simulink model "MSBR_Plant"  (R2021b)
settings: Solver=ode45  StartTime=0.0  StopTime=sim_time  MaxStep=ts_max  RelTol=1e-4
values from neighbouring files (symbols this model uses):
  a_1 = 8.7292e-2/wilson_ratio    (= 0.0087292)    [Whole_Plant_Cool_Pump_Accident_script.m]    (also in Whole_Plant_Fert_Pump_Accident_script.m; Whole_Plant_Fuel_Pump_Accident.m; Whole_Plant_Fuel_Pump_Accident_script.m; Whole_Plant_Reactivity_Accident.m)
  a_2 = 7.3787e-4/wilson_ratio    (= 7.3787e-05)    [Whole_Plant_Cool_Pump_Accident_script.m]    (also in Whole_Plant_Fert_Pump_Accident_script.m; Whole_Plant_Fuel_Pump_Accident.m; Whole_Plant_Fuel_Pump_Accident_script.m; Whole_Plant_Reactivity_Accident.m)
  a_b = 1.656e-5    (= 1.656e-05)    [Whole_Plant_Cool_Pump_Accident_script.m]    (also in Whole_Plant_Fert_Pump_Accident_script.m; Whole_Plant_Fuel_Pump_Accident.m; Whole_Plant_Fuel_Pump_Accident_script.m; Whole_Plant_Reactivity_Accident.m)
  a_f = -8.172e-5    (= -8.172e-05)    [Whole_Plant_Cool_Pump_Accident_script.m]    (also in Whole_Plant_Fert_Pump_Accident_script.m; Whole_Plant_Fuel_Pump_Accident.m; Whole_Plant_Fuel_Pump_Accident_script.m; Whole_Plant_Reactivity_Accident.m)
  a_g = 2.016e-5    (= 2.016e-05)    [Whole_Plant_Cool_Pump_Accident_script.m]    (also in Whole_Plant_Fert_Pump_Accident_script.m; Whole_Plant_Fuel_Pump_Accident.m; Whole_Plant_Fuel_Pump_Accident_script.m; Whole_Plant_Reactivity_Accident.m)
  A_s = pi()*((D_OTSG_i^2)/4) - A_w_OTSG - A_p_OTSG    [Whole_Plant_Cool_Pump_Accident_script.m]    (also in Whole_Plant_Fert_Pump_Accident_script.m; Whole_Plant_Fuel_Pump_Accident.m; Whole_Plant_Fuel_Pump_Accident_script.m; Whole_Plant_Reactivity_Accident.m)
  alpha_co = 316.2    [Whole_Plant_Cool_Pump_Accident_script.m]    (also in Whole_Plant_Fert_Pump_Accident_script.m; Whole_Plant_Fuel_Pump_Accident.m; Whole_Plant_Fuel_Pump_Accident_script.m; Whole_Plant_Reactivity_Accident.m)
  beta = [2.290e-04, 8.320e-04, 7.100e-04, 8.520e-04, 1.710e-04, 1.020e-04]    [Whole_Plant_Cool_Pump_Accident_script.m]    (also in Whole_Plant_Fert_Pump_Accident_script.m; Whole_Plant_Fuel_Pump_Accident.m; Whole_Plant_Fuel_Pump_Accident_script.m; Whole_Plant_Reactivity_Accident.m)
  beta_co = 68.0958    [Whole_Plant_Cool_Pump_Accident_script.m]    (also in Whole_Plant_Fert_Pump_Accident_script.m; Whole_Plant_Fuel_Pump_Accident.m; Whole_Plant_Fuel_Pump_Accident_script.m; Whole_Plant_Reactivity_Accident.m)
  beta_t = sum(beta)    [Whole_Plant_Cool_Pump_Accident_script.m]    (also in Whole_Plant_Fert_Pump_Accident_script.m; Whole_Plant_Fuel_Pump_Accident.m; Whole_Plant_Fuel_Pump_Accident_script.m; Whole_Plant_Reactivity_Accident.m)
  C_nc_X_A_nc = 12.8    [Whole_Plant_Cool_Pump_Accident_script.m]    (also in Whole_Plant_Fert_Pump_Accident_script.m; Whole_Plant_Fuel_Pump_Accident.m; Whole_Plant_Fuel_Pump_Accident_script.m; Whole_Plant_Reactivity_Accident.m)
  C_pcw = 0.0042    [Whole_Plant_Cool_Pump_Accident_script.m]    (also in Whole_Plant_Fert_Pump_Accident_script.m; Whole_Plant_Fuel_Pump_Accident.m; Whole_Plant_Fuel_Pump_Accident_script.m; Whole_Plant_Reactivity_Accident.m)
  C_rh_X_A_rh = 33    [Whole_Plant_Cool_Pump_Accident_script.m]    (also in Whole_Plant_Fert_Pump_Accident_script.m; Whole_Plant_Fuel_Pump_Accident.m; Whole_Plant_Fuel_Pump_Accident_script.m; Whole_Plant_Reactivity_Accident.m)
  C_v = 0.84    [Whole_Plant_Cool_Pump_Accident_script.m]    (also in Whole_Plant_Fert_Pump_Accident_script.m; Whole_Plant_Fuel_Pump_Accident.m; Whole_Plant_Fuel_Pump_Accident_script.m; Whole_Plant_Reactivity_Accident.m)
  ce1 = 1.2471e-07    [Whole_Plant_Cool_Pump_Accident_script.m]    (also in Whole_Plant_Fert_Pump_Accident_script.m; Whole_Plant_Fuel_Pump_Accident.m; Whole_Plant_Fuel_Pump_Accident_script.m; Whole_Plant_Reactivity_Accident.m)
  ce2 = 5.3816e-14    [Whole_Plant_Cool_Pump_Accident_script.m]    (also in Whole_Plant_Fert_Pump_Accident_script.m; Whole_Plant_Fuel_Pump_Accident.m; Whole_Plant_Fuel_Pump_Accident_script.m; Whole_Plant_Reactivity_Accident.m)
  ce3 = 3.3721e-08    [Whole_Plant_Cool_Pump_Accident_script.m]    (also in Whole_Plant_Fert_Pump_Accident_script.m; Whole_Plant_Fuel_Pump_Accident.m; Whole_Plant_Fuel_Pump_Accident_script.m; Whole_Plant_Reactivity_Accident.m)
  Cp_fw = XSteam('Cp_pT',P_set*10,T_fw)/1000    [Whole_Plant_Cool_Pump_Accident_script.m]    (also in Whole_Plant_Fert_Pump_Accident_script.m; Whole_Plant_Fuel_Pump_Accident.m; Whole_Plant_Fuel_Pump_Accident_script.m; Whole_Plant_Reactivity_Accident.m)
  Cp_p = Cp_sec    (= 0.001716588)    [Whole_Plant_Cool_Pump_Accident_script.m]    (also in Whole_Plant_Fert_Pump_Accident_script.m; Whole_Plant_Fuel_Pump_Accident.m; Whole_Plant_Fuel_Pump_Accident_script.m; Whole_Plant_Reactivity_Accident.m)
  Cp_rh = 0.0021520    (= 0.002152)    [Whole_Plant_Cool_Pump_Accident_script.m]    (also in Whole_Plant_Fert_Pump_Accident_script.m; Whole_Plant_Fuel_Pump_Accident.m; Whole_Plant_Fuel_Pump_Accident_script.m; Whole_Plant_Reactivity_Accident.m)
  Cp_s = XSteam('Cp_pT',P_s*10,T_s)/1000    [Whole_Plant_Cool_Pump_Accident_script.m]    (also in Whole_Plant_Fert_Pump_Accident_script.m; Whole_Plant_Fuel_Pump_Accident.m; Whole_Plant_Fuel_Pump_Accident_script.m; Whole_Plant_Reactivity_Accident.m)
  Cp_sc = XSteam('Cp_pT',P_set*10,T_sc2)/1000    [Whole_Plant_Cool_Pump_Accident_script.m]    (also in Whole_Plant_Fert_Pump_Accident_script.m; Whole_Plant_Fuel_Pump_Accident.m; Whole_Plant_Fuel_Pump_Accident_script.m; Whole_Plant_Reactivity_Accident.m)
  Cp_w = 468.992e-6    (= 0.000468992)    [Whole_Plant_Cool_Pump_Accident_script.m]    (also in Whole_Plant_Fert_Pump_Accident_script.m; Whole_Plant_Fuel_Pump_Accident.m; Whole_Plant_Fuel_Pump_Accident_script.m; Whole_Plant_Reactivity_Accident.m)
  D_it = D_ot-2*T_th    (= 0.014147)    [Whole_Plant_Cool_Pump_Accident_script.m]    (also in Whole_Plant_Fert_Pump_Accident_script.m; Whole_Plant_Fuel_Pump_Accident.m; Whole_Plant_Fuel_Pump_Accident_script.m; Whole_Plant_Reactivity_Accident.m)
  D_ot = 0.015875    [Whole_Plant_Cool_Pump_Accident_script.m]    (also in Whole_Plant_Fert_Pump_Accident_script.m; Whole_Plant_Fuel_Pump_Accident.m; Whole_Plant_Fuel_Pump_Accident_script.m; Whole_Plant_Reactivity_Accident.m)
  dHs_dPs = c(1)    [Whole_Plant_Cool_Pump_Accident_script.m]    (also in Whole_Plant_Fert_Pump_Accident_script.m; Whole_Plant_Fuel_Pump_Accident.m; Whole_Plant_Fuel_Pump_Accident_script.m; Whole_Plant_Reactivity_Accident.m)
  eta_hp_isen = 0.861    [Whole_Plant_Cool_Pump_Accident_script.m]    (also in Whole_Plant_Fert_Pump_Accident_script.m; Whole_Plant_Fuel_Pump_Accident.m; Whole_Plant_Fuel_Pump_Accident_script.m; Whole_Plant_Reactivity_Accident.m)
  eta_lp_isen = 0.861    [Whole_Plant_Cool_Pump_Accident_script.m]    (also in Whole_Plant_Fert_Pump_Accident_script.m; Whole_Plant_Fuel_Pump_Accident.m; Whole_Plant_Fuel_Pump_Accident_script.m; Whole_Plant_Reactivity_Accident.m)
  gamma_I = 5.1135e-2    (= 0.051135)    [Whole_Plant_Cool_Pump_Accident_script.m]    (also in Whole_Plant_Fert_Pump_Accident_script.m; Whole_Plant_Fuel_Pump_Accident.m; Whole_Plant_Fuel_Pump_Accident_script.m; Whole_Plant_Reactivity_Accident.m)
  gamma_Xe = 1.1628e-2    (= 0.011628)    [Whole_Plant_Cool_Pump_Accident_script.m]    (also in Whole_Plant_Fert_Pump_Accident_script.m; Whole_Plant_Fuel_Pump_Accident.m; Whole_Plant_Fuel_Pump_Accident_script.m; Whole_Plant_Reactivity_Accident.m)
  H_co0 = 0.149    [Whole_Plant_Cool_Pump_Accident_script.m]    (also in Whole_Plant_Fert_Pump_Accident_script.m; Whole_Plant_Fuel_Pump_Accident.m; Whole_Plant_Fuel_Pump_Accident_script.m; Whole_Plant_Reactivity_Accident.m)
  H_f_co0 = 0.149    [Whole_Plant_Cool_Pump_Accident_script.m]    (also in Whole_Plant_Fert_Pump_Accident_script.m; Whole_Plant_Fuel_Pump_Accident.m; Whole_Plant_Fuel_Pump_Accident_script.m; Whole_Plant_Reactivity_Accident.m)
  H_fg_co0 = 2.35    [Whole_Plant_Cool_Pump_Accident_script.m]    (also in Whole_Plant_Fert_Pump_Accident_script.m; Whole_Plant_Fuel_Pump_Accident.m; Whole_Plant_Fuel_Pump_Accident_script.m; Whole_Plant_Reactivity_Accident.m)
  H_fgrh0 = (XSteam('hV_p', P_s*1e1) - XSteam('hL_p', P_s*1e1))/1e3    [Whole_Plant_Cool_Pump_Accident_script.m]    (also in Whole_Plant_Fert_Pump_Accident_script.m; Whole_Plant_Fuel_Pump_Accident.m; Whole_Plant_Fuel_Pump_Accident_script.m; Whole_Plant_Reactivity_Accident.m)
  H_frh0 = XSteam('hL_p', P_s*1e1)/1e3    [Whole_Plant_Cool_Pump_Accident_script.m]    (also in Whole_Plant_Fert_Pump_Accident_script.m; Whole_Plant_Fuel_Pump_Accident.m; Whole_Plant_Fuel_Pump_Accident_script.m; Whole_Plant_Reactivity_Accident.m)
  h_fwh1 = 0.5927    [Whole_Plant_Cool_Pump_Accident_script.m]    (also in Whole_Plant_Fert_Pump_Accident_script.m; Whole_Plant_Fuel_Pump_Accident.m; Whole_Plant_Fuel_Pump_Accident_script.m; Whole_Plant_Reactivity_Accident.m)
  H_fwh10 = 0.46009    [Whole_Plant_Cool_Pump_Accident_script.m]    (also in Whole_Plant_Fert_Pump_Accident_script.m; Whole_Plant_Fuel_Pump_Accident.m; Whole_Plant_Fuel_Pump_Accident_script.m; Whole_Plant_Reactivity_Accident.m)
  h_fwh2 = 1.230803    [Whole_Plant_Cool_Pump_Accident_script.m]    (also in Whole_Plant_Fert_Pump_Accident_script.m; Whole_Plant_Fuel_Pump_Accident.m; Whole_Plant_Fuel_Pump_Accident_script.m; Whole_Plant_Reactivity_Accident.m)
  H_fwh20 = 0.6784    [Whole_Plant_Cool_Pump_Accident_script.m]    (also in Whole_Plant_Fert_Pump_Accident_script.m; Whole_Plant_Fuel_Pump_Accident.m; Whole_Plant_Fuel_Pump_Accident_script.m; Whole_Plant_Reactivity_Accident.m)
  H_grh0 = 2.8029    [Whole_Plant_Cool_Pump_Accident_script.m]    (also in Whole_Plant_Fert_Pump_Accident_script.m; Whole_Plant_Fuel_Pump_Accident.m; Whole_Plant_Fuel_Pump_Accident_script.m; Whole_Plant_Reactivity_Accident.m)
  H_hp_isen0 = 2.5111    [Whole_Plant_Cool_Pump_Accident_script.m]    (also in Whole_Plant_Fert_Pump_Accident_script.m; Whole_Plant_Fuel_Pump_Accident.m; Whole_Plant_Fuel_Pump_Accident_script.m; Whole_Plant_Reactivity_Accident.m)
  H_hpt_out = 2.6201    [Whole_Plant_Cool_Pump_Accident_script.m]    (also in Whole_Plant_Fert_Pump_Accident_script.m; Whole_Plant_Fuel_Pump_Accident.m; Whole_Plant_Fuel_Pump_Accident_script.m; Whole_Plant_Reactivity_Accident.m)
  H_lp_isen = 958.4*1054.35e-6/0.45359237    (= 2.22774699671)    [Whole_Plant_Cool_Pump_Accident_script.m]    (also in Whole_Plant_Fert_Pump_Accident_script.m; Whole_Plant_Fuel_Pump_Accident.m; Whole_Plant_Fuel_Pump_Accident_script.m; Whole_Plant_Reactivity_Accident.m)
  H_lpt_out = 2.3089    [Whole_Plant_Cool_Pump_Accident_script.m]    (also in Whole_Plant_Fert_Pump_Accident_script.m; Whole_Plant_Fuel_Pump_Accident.m; Whole_Plant_Fuel_Pump_Accident_script.m; Whole_Plant_Reactivity_Accident.m)
  H_nc = XSteam('h_pT', P_s*10, T_s)/1000    [Whole_Plant_Cool_Pump_Accident_script.m]    (also in Whole_Plant_Fert_Pump_Accident_script.m; Whole_Plant_Fuel_Pump_Accident.m; Whole_Plant_Fuel_Pump_Accident_script.m; Whole_Plant_Reactivity_Accident.m)
  h_pw = h_s    (= 0.02555)    [Whole_Plant_Cool_Pump_Accident_script.m]    (also in Whole_Plant_Fert_Pump_Accident_script.m; Whole_Plant_Fuel_Pump_Accident.m; Whole_Plant_Fuel_Pump_Accident_script.m; Whole_Plant_Reactivity_Accident.m)
  H_rh = 2.8115    [Whole_Plant_Cool_Pump_Accident_script.m]    (also in Whole_Plant_Fert_Pump_Accident_script.m; Whole_Plant_Fuel_Pump_Accident.m; Whole_Plant_Fuel_Pump_Accident_script.m; Whole_Plant_Reactivity_Accident.m)
  h_wb = 13349.334646671E-6    (= 0.0133493346467)    [Whole_Plant_Cool_Pump_Accident_script.m]    (also in Whole_Plant_Fert_Pump_Accident_script.m; Whole_Plant_Fuel_Pump_Accident.m; Whole_Plant_Fuel_Pump_Accident_script.m; Whole_Plant_Reactivity_Accident.m)
  h_ws = 5732.378387768E-6    (= 0.00573237838777)    [Whole_Plant_Cool_Pump_Accident_script.m]    (also in Whole_Plant_Fert_Pump_Accident_script.m; Whole_Plant_Fuel_Pump_Accident.m; Whole_Plant_Fuel_Pump_Accident_script.m; Whole_Plant_Reactivity_Accident.m)
  h_wsc = 8385.005556375E-6    (= 0.00838500555638)    [Whole_Plant_Cool_Pump_Accident_script.m]    (also in Whole_Plant_Fert_Pump_Accident_script.m; Whole_Plant_Fuel_Pump_Accident.m; Whole_Plant_Fuel_Pump_Accident_script.m; Whole_Plant_Reactivity_Accident.m)
  hA_bg = A_fert*h_bg    (= 2.76411813627)    [Whole_Plant_Cool_Pump_Accident_script.m]    (also in Whole_Plant_Fert_Pump_Accident_script.m; Whole_Plant_Fuel_Pump_Accident.m; Whole_Plant_Fuel_Pump_Accident_script.m; Whole_Plant_Reactivity_Accident.m)
  hA_co0 = 140    [Whole_Plant_Cool_Pump_Accident_script.m]    (also in Whole_Plant_Fert_Pump_Accident_script.m; Whole_Plant_Fuel_Pump_Accident.m; Whole_Plant_Fuel_Pump_Accident_script.m; Whole_Plant_Reactivity_Accident.m)
  hA_fg_dn = h_fg*A_fuel_down    [Whole_Plant_Cool_Pump_Accident_script.m]    (also in Whole_Plant_Fert_Pump_Accident_script.m; Whole_Plant_Fuel_Pump_Accident.m; Whole_Plant_Fuel_Pump_Accident_script.m; Whole_Plant_Reactivity_Accident.m)
  hA_fg_up = h_fg*A_fuel_up    [Whole_Plant_Cool_Pump_Accident_script.m]    (also in Whole_Plant_Fert_Pump_Accident_script.m; Whole_Plant_Fuel_Pump_Accident.m; Whole_Plant_Fuel_Pump_Accident_script.m; Whole_Plant_Reactivity_Accident.m)
  hA_p_bhx1 = [h_pb*A_pbhx/2,h_pb*A_pbhx/2]    [Whole_Plant_Cool_Pump_Accident_script.m]    (also in Whole_Plant_Fert_Pump_Accident_script.m; Whole_Plant_Fuel_Pump_Accident.m; Whole_Plant_Fuel_Pump_Accident_script.m; Whole_Plant_Reactivity_Accident.m)
  hA_p_bhx2 = hA_p_bhx1    [Whole_Plant_Cool_Pump_Accident_script.m]    (also in Whole_Plant_Fert_Pump_Accident_script.m; Whole_Plant_Fuel_Pump_Accident.m; Whole_Plant_Fuel_Pump_Accident_script.m; Whole_Plant_Reactivity_Accident.m)
  hA_p_bhx3 = hA_p_bhx1    [Whole_Plant_Cool_Pump_Accident_script.m]    (also in Whole_Plant_Fert_Pump_Accident_script.m; Whole_Plant_Fuel_Pump_Accident.m; Whole_Plant_Fuel_Pump_Accident_script.m; Whole_Plant_Reactivity_Accident.m)
  hA_p_bhx4 = hA_p_bhx1    [Whole_Plant_Cool_Pump_Accident_script.m]    (also in Whole_Plant_Fert_Pump_Accident_script.m; Whole_Plant_Fuel_Pump_Accident.m; Whole_Plant_Fuel_Pump_Accident_script.m; Whole_Plant_Reactivity_Accident.m)
  hA_p_fhx1 = [h_p*A_pfhx_dn/2,h_p*A_pfhx_dn/2,h_p*A_pfhx_up/2,h_p*A_pfhx_up/2]    [Whole_Plant_Cool_Pump_Accident_script.m]    (also in Whole_Plant_Fert_Pump_Accident_script.m; Whole_Plant_Fuel_Pump_Accident.m; Whole_Plant_Fuel_Pump_Accident_script.m; Whole_Plant_Reactivity_Accident.m)
  hA_p_fhx2 = hA_p_fhx1    [Whole_Plant_Cool_Pump_Accident_script.m]    (also in Whole_Plant_Fert_Pump_Accident_script.m; Whole_Plant_Fuel_Pump_Accident.m; Whole_Plant_Fuel_Pump_Accident_script.m; Whole_Plant_Reactivity_Accident.m)
  hA_p_fhx3 = hA_p_fhx1    [Whole_Plant_Cool_Pump_Accident_script.m]    (also in Whole_Plant_Fert_Pump_Accident_script.m; Whole_Plant_Fuel_Pump_Accident.m; Whole_Plant_Fuel_Pump_Accident_script.m; Whole_Plant_Reactivity_Accident.m)
  hA_p_fhx4 = hA_p_fhx1    [Whole_Plant_Cool_Pump_Accident_script.m]    (also in Whole_Plant_Fert_Pump_Accident_script.m; Whole_Plant_Fuel_Pump_Accident.m; Whole_Plant_Fuel_Pump_Accident_script.m; Whole_Plant_Reactivity_Accident.m)
  hA_s_bhx1 = [h_sb*A_sbhx/2,h_sb*A_sbhx/2]    [Whole_Plant_Cool_Pump_Accident_script.m]    (also in Whole_Plant_Fert_Pump_Accident_script.m; Whole_Plant_Fuel_Pump_Accident.m; Whole_Plant_Fuel_Pump_Accident_script.m; Whole_Plant_Reactivity_Accident.m)
  hA_s_bhx2 = hA_s_bhx1    [Whole_Plant_Cool_Pump_Accident_script.m]    (also in Whole_Plant_Fert_Pump_Accident_script.m; Whole_Plant_Fuel_Pump_Accident.m; Whole_Plant_Fuel_Pump_Accident_script.m; Whole_Plant_Reactivity_Accident.m)
  hA_s_bhx3 = hA_s_bhx1    [Whole_Plant_Cool_Pump_Accident_script.m]    (also in Whole_Plant_Fert_Pump_Accident_script.m; Whole_Plant_Fuel_Pump_Accident.m; Whole_Plant_Fuel_Pump_Accident_script.m; Whole_Plant_Reactivity_Accident.m)
  hA_s_bhx4 = hA_s_bhx1    [Whole_Plant_Cool_Pump_Accident_script.m]    (also in Whole_Plant_Fert_Pump_Accident_script.m; Whole_Plant_Fuel_Pump_Accident.m; Whole_Plant_Fuel_Pump_Accident_script.m; Whole_Plant_Reactivity_Accident.m)
  hA_s_fhx1 = [h_s*A_sfhx_up/2,h_s*A_sfhx_up/2,h_s*A_sfhx_dn/2,h_s*A_sfhx_dn/2]    [Whole_Plant_Cool_Pump_Accident_script.m]    (also in Whole_Plant_Fert_Pump_Accident_script.m; Whole_Plant_Fuel_Pump_Accident.m; Whole_Plant_Fuel_Pump_Accident_script.m; Whole_Plant_Reactivity_Accident.m)
  hA_s_fhx2 = hA_s_fhx1    [Whole_Plant_Cool_Pump_Accident_script.m]    (also in Whole_Plant_Fert_Pump_Accident_script.m; Whole_Plant_Fuel_Pump_Accident.m; Whole_Plant_Fuel_Pump_Accident_script.m; Whole_Plant_Reactivity_Accident.m)
  hA_s_fhx3 = hA_s_fhx1    [Whole_Plant_Cool_Pump_Accident_script.m]    (also in Whole_Plant_Fert_Pump_Accident_script.m; Whole_Plant_Fuel_Pump_Accident.m; Whole_Plant_Fuel_Pump_Accident_script.m; Whole_Plant_Reactivity_Accident.m)
  hA_s_fhx4 = hA_s_fhx1    [Whole_Plant_Cool_Pump_Accident_script.m]    (also in Whole_Plant_Fert_Pump_Accident_script.m; Whole_Plant_Fuel_Pump_Accident.m; Whole_Plant_Fuel_Pump_Accident_script.m; Whole_Plant_Reactivity_Accident.m)
  I_0 = gamma_I*Sigma_f_msbr*phi_0/lam_I    (= 1.30000734126e+17)    [Whole_Plant_Cool_Pump_Accident_script.m]    (also in Whole_Plant_Fert_Pump_Accident_script.m; Whole_Plant_Fuel_Pump_Accident.m; Whole_Plant_Fuel_Pump_Accident_script.m; Whole_Plant_Reactivity_Accident.m)
  k_1 = 0.5    [Whole_Plant_Cool_Pump_Accident_script.m]    (also in Whole_Plant_Fert_Pump_Accident_script.m; Whole_Plant_Fuel_Pump_Accident.m; Whole_Plant_Fuel_Pump_Accident_script.m; Whole_Plant_Reactivity_Accident.m)
  K_1 = e(1)    [Whole_Plant_Cool_Pump_Accident_script.m]    (also in Whole_Plant_Fert_Pump_Accident_script.m; Whole_Plant_Fuel_Pump_Accident.m; Whole_Plant_Fuel_Pump_Accident_script.m; Whole_Plant_Reactivity_Accident.m)
  k_1b = 0.5    [Whole_Plant_Cool_Pump_Accident_script.m]    (also in Whole_Plant_Fert_Pump_Accident_script.m; Whole_Plant_Fuel_Pump_Accident.m; Whole_Plant_Fuel_Pump_Accident_script.m; Whole_Plant_Reactivity_Accident.m)
  k_2 = 0.5    [Whole_Plant_Cool_Pump_Accident_script.m]    (also in Whole_Plant_Fert_Pump_Accident_script.m; Whole_Plant_Fuel_Pump_Accident.m; Whole_Plant_Fuel_Pump_Accident_script.m; Whole_Plant_Reactivity_Accident.m)
  k_2b = 0.5    [Whole_Plant_Cool_Pump_Accident_script.m]    (also in Whole_Plant_Fert_Pump_Accident_script.m; Whole_Plant_Fuel_Pump_Accident.m; Whole_Plant_Fuel_Pump_Accident_script.m; Whole_Plant_Reactivity_Accident.m)
  k_3 = 0.5    [Whole_Plant_Cool_Pump_Accident_script.m]    (also in Whole_Plant_Fert_Pump_Accident_script.m; Whole_Plant_Fuel_Pump_Accident.m; Whole_Plant_Fuel_Pump_Accident_script.m; Whole_Plant_Reactivity_Accident.m)
  k_4 = 0.5    [Whole_Plant_Cool_Pump_Accident_script.m]    (also in Whole_Plant_Fert_Pump_Accident_script.m; Whole_Plant_Fuel_Pump_Accident.m; Whole_Plant_Fuel_Pump_Accident_script.m; Whole_Plant_Reactivity_Accident.m)
  K_4 = b(1)    [Whole_Plant_Cool_Pump_Accident_script.m]    (also in Whole_Plant_Fert_Pump_Accident_script.m; Whole_Plant_Fuel_Pump_Accident.m; Whole_Plant_Fuel_Pump_Accident_script.m; Whole_Plant_Reactivity_Accident.m)
  K_5 = a(1)    [Whole_Plant_Cool_Pump_Accident_script.m]    (also in Whole_Plant_Fert_Pump_Accident_script.m; Whole_Plant_Fuel_Pump_Accident.m; Whole_Plant_Fuel_Pump_Accident_script.m; Whole_Plant_Reactivity_Accident.m)
  K_b = d(1)    [Whole_Plant_Cool_Pump_Accident_script.m]    (also in Whole_Plant_Fert_Pump_Accident_script.m; Whole_Plant_Fuel_Pump_Accident.m; Whole_Plant_Fuel_Pump_Accident_script.m; Whole_Plant_Reactivity_Accident.m)
  k_b1 = (K_B/2)/K    (= 0.0089463103122)    [Whole_Plant_Cool_Pump_Accident_script.m]    (also in Whole_Plant_Fert_Pump_Accident_script.m; Whole_Plant_Fuel_Pump_Accident.m; Whole_Plant_Fuel_Pump_Accident_script.m; Whole_Plant_Reactivity_Accident.m)
  k_b2 = k_b1    (= 0.0089463103122)    [Whole_Plant_Cool_Pump_Accident_script.m]    (also in Whole_Plant_Fert_Pump_Accident_script.m; Whole_Plant_Fuel_Pump_Accident.m; Whole_Plant_Fuel_Pump_Accident_script.m; Whole_Plant_Reactivity_Accident.m)
  K_bhp = 0.1634    [Whole_Plant_Cool_Pump_Accident_script.m]    (also in Whole_Plant_Fert_Pump_Accident_script.m; Whole_Plant_Fuel_Pump_Accident.m; Whole_Plant_Fuel_Pump_Accident_script.m; Whole_Plant_Reactivity_Accident.m)
  K_blp = 0.2174    [Whole_Plant_Cool_Pump_Accident_script.m]    (also in Whole_Plant_Fert_Pump_Accident_script.m; Whole_Plant_Fuel_Pump_Accident.m; Whole_Plant_Fuel_Pump_Accident_script.m; Whole_Plant_Reactivity_Accident.m)
  k_f1 = ((1 - K_G - K_B - K_Ba)/4)/K    (= 0.226055463576)    [Whole_Plant_Cool_Pump_Accident_script.m]    (also in Whole_Plant_Fert_Pump_Accident_script.m; Whole_Plant_Fuel_Pump_Accident.m; Whole_Plant_Fuel_Pump_Accident_script.m; Whole_Plant_Reactivity_Accident.m)
  k_f2 = k_f1    (= 0.226055463576)    [Whole_Plant_Cool_Pump_Accident_script.m]    (also in Whole_Plant_Fert_Pump_Accident_script.m; Whole_Plant_Fuel_Pump_Accident.m; Whole_Plant_Fuel_Pump_Accident_script.m; Whole_Plant_Reactivity_Accident.m)
  k_f3 = k_f1    (= 0.226055463576)    [Whole_Plant_Cool_Pump_Accident_script.m]    (also in Whole_Plant_Fert_Pump_Accident_script.m; Whole_Plant_Fuel_Pump_Accident.m; Whole_Plant_Fuel_Pump_Accident_script.m; Whole_Plant_Reactivity_Accident.m)
  k_f4 = k_f1    (= 0.226055463576)    [Whole_Plant_Cool_Pump_Accident_script.m]    (also in Whole_Plant_Fert_Pump_Accident_script.m; Whole_Plant_Fuel_Pump_Accident.m; Whole_Plant_Fuel_Pump_Accident_script.m; Whole_Plant_Reactivity_Accident.m)
  k_g1 = ((K_G*K_fuel)/2)/K    (= 0.0346590586566)    [Whole_Plant_Cool_Pump_Accident_script.m]    (also in Whole_Plant_Fert_Pump_Accident_script.m; Whole_Plant_Fuel_Pump_Accident.m; Whole_Plant_Fuel_Pump_Accident_script.m; Whole_Plant_Reactivity_Accident.m)
  k_g2 = k_g1    (= 0.0346590586566)    [Whole_Plant_Cool_Pump_Accident_script.m]    (also in Whole_Plant_Fert_Pump_Accident_script.m; Whole_Plant_Fuel_Pump_Accident.m; Whole_Plant_Fuel_Pump_Accident_script.m; Whole_Plant_Reactivity_Accident.m)
  k_g3 = (K_G*(1-K_fuel))/K    (= 0.00856740775781)    [Whole_Plant_Cool_Pump_Accident_script.m]    (also in Whole_Plant_Fert_Pump_Accident_script.m; Whole_Plant_Fuel_Pump_Accident.m; Whole_Plant_Fuel_Pump_Accident_script.m; Whole_Plant_Reactivity_Accident.m)
  K_sc = f(1)    [Whole_Plant_Cool_Pump_Accident_script.m]    (also in Whole_Plant_Fert_Pump_Accident_script.m; Whole_Plant_Fuel_Pump_Accident.m; Whole_Plant_Fuel_Pump_Accident_script.m; Whole_Plant_Reactivity_Accident.m)
  L = 22.0    (= 22)    [Whole_Plant_Cool_Pump_Accident_script.m]    (also in Whole_Plant_Fert_Pump_Accident_script.m; Whole_Plant_Fuel_Pump_Accident.m; Whole_Plant_Fuel_Pump_Accident_script.m; Whole_Plant_Reactivity_Accident.m)
  L_b = 1.9    [Whole_Plant_Cool_Pump_Accident_script.m]    (also in Whole_Plant_Fert_Pump_Accident_script.m; Whole_Plant_Fuel_Pump_Accident.m; Whole_Plant_Fuel_Pump_Accident_script.m; Whole_Plant_Reactivity_Accident.m)
  L_s = 16.53    [Whole_Plant_Cool_Pump_Accident_script.m]    (also in Whole_Plant_Fert_Pump_Accident_script.m; Whole_Plant_Fuel_Pump_Accident.m; Whole_Plant_Fuel_Pump_Accident_script.m; Whole_Plant_Reactivity_Accident.m)
  L_sc = L-L_b-L_s    (= 3.57)    [Whole_Plant_Cool_Pump_Accident_script.m]    (also in Whole_Plant_Fert_Pump_Accident_script.m; Whole_Plant_Fuel_Pump_Accident.m; Whole_Plant_Fuel_Pump_Accident_script.m; Whole_Plant_Reactivity_Accident.m)
  Lam = 3.3e-4    (= 0.00033)    [Whole_Plant_Cool_Pump_Accident_script.m]    (also in Whole_Plant_Fert_Pump_Accident_script.m; Whole_Plant_Fuel_Pump_Accident.m; Whole_Plant_Fuel_Pump_Accident_script.m; Whole_Plant_Reactivity_Accident.m)
  lam = [1.260e-02, 3.370e-02, 1.390e-01, 3.250e-01, 1.130e+00, 2.500e+00]    [Whole_Plant_Cool_Pump_Accident_script.m]    (also in Whole_Plant_Fert_Pump_Accident_script.m; Whole_Plant_Fuel_Pump_Accident.m; Whole_Plant_Fuel_Pump_Accident_script.m; Whole_Plant_Reactivity_Accident.m)
  lam_bubl = 2.0e-2    (= 0.02)    [Whole_Plant_Cool_Pump_Accident_script.m]    (also in Whole_Plant_Fert_Pump_Accident_script.m; Whole_Plant_Fuel_Pump_Accident.m; Whole_Plant_Fuel_Pump_Accident_script.m; Whole_Plant_Reactivity_Accident.m)
  lam_I = 2.875e-5    (= 2.875e-05)    [Whole_Plant_Cool_Pump_Accident_script.m]    (also in Whole_Plant_Fert_Pump_Accident_script.m; Whole_Plant_Fuel_Pump_Accident.m; Whole_Plant_Fuel_Pump_Accident_script.m; Whole_Plant_Reactivity_Accident.m)
  lam_Xe = 2.0916e-5    (= 2.0916e-05)    [Whole_Plant_Cool_Pump_Accident_script.m]    (also in Whole_Plant_Fert_Pump_Accident_script.m; Whole_Plant_Fuel_Pump_Accident.m; Whole_Plant_Fuel_Pump_Accident_script.m; Whole_Plant_Reactivity_Accident.m)
  m_bm = (W_b1+W_b2+W_b3+W_b4)*time_mixb    (= 2167.1636)    [Whole_Plant_Cool_Pump_Accident_script.m]    (also in Whole_Plant_Fert_Pump_Accident_script.m; Whole_Plant_Fuel_Pump_Accident.m; Whole_Plant_Fuel_Pump_Accident_script.m; Whole_Plant_Reactivity_Accident.m)
  M_cw = 65000    [Whole_Plant_Cool_Pump_Accident_script.m]    (also in Whole_Plant_Fert_Pump_Accident_script.m; Whole_Plant_Fuel_Pump_Accident.m; Whole_Plant_Fuel_Pump_Accident_script.m; Whole_Plant_Reactivity_Accident.m)
  m_fm = (W_f1+W_f2+W_f3+W_f4)*time_mixf    (= 5443.108)    [Whole_Plant_Cool_Pump_Accident_script.m]    (also in Whole_Plant_Fert_Pump_Accident_script.m; Whole_Plant_Fuel_Pump_Accident.m; Whole_Plant_Fuel_Pump_Accident_script.m; Whole_Plant_Reactivity_Accident.m)
  M_hw0 = 10000    [Whole_Plant_Cool_Pump_Accident_script.m]    (also in Whole_Plant_Fert_Pump_Accident_script.m; Whole_Plant_Fuel_Pump_Accident.m; Whole_Plant_Fuel_Pump_Accident_script.m; Whole_Plant_Reactivity_Accident.m)
  m_sm = (W_s1+W_s2+W_s3+W_s4)*time_mixs    (= 8467.056)    [Whole_Plant_Cool_Pump_Accident_script.m]    (also in Whole_Plant_Fert_Pump_Accident_script.m; Whole_Plant_Fuel_Pump_Accident.m; Whole_Plant_Fuel_Pump_Accident_script.m; Whole_Plant_Reactivity_Accident.m)
  M_stm = 0.018    [Whole_Plant_Cool_Pump_Accident_script.m]    (also in Whole_Plant_Fert_Pump_Accident_script.m; Whole_Plant_Fuel_Pump_Accident.m; Whole_Plant_Fuel_Pump_Accident_script.m; Whole_Plant_Reactivity_Accident.m)
  mcp_b1 = mass_bn*Cp_b    (= 4.17494922705)    [Whole_Plant_Cool_Pump_Accident_script.m]    (also in Whole_Plant_Fert_Pump_Accident_script.m; Whole_Plant_Fuel_Pump_Accident.m; Whole_Plant_Fuel_Pump_Accident_script.m; Whole_Plant_Reactivity_Accident.m)
  mcp_b2 = mcp_b1    (= 4.17494922705)    [Whole_Plant_Cool_Pump_Accident_script.m]    (also in Whole_Plant_Fert_Pump_Accident_script.m; Whole_Plant_Fuel_Pump_Accident.m; Whole_Plant_Fuel_Pump_Accident_script.m; Whole_Plant_Reactivity_Accident.m)
  mcp_f1 = mass_fn*Cp_f    (= 5.5019469141)    [Whole_Plant_Cool_Pump_Accident_script.m]    (also in Whole_Plant_Fert_Pump_Accident_script.m; Whole_Plant_Fuel_Pump_Accident.m; Whole_Plant_Fuel_Pump_Accident_script.m; Whole_Plant_Reactivity_Accident.m)
  mcp_f2 = mass_fn*Cp_f    (= 5.5019469141)    [Whole_Plant_Cool_Pump_Accident_script.m]    (also in Whole_Plant_Fert_Pump_Accident_script.m; Whole_Plant_Fuel_Pump_Accident.m; Whole_Plant_Fuel_Pump_Accident_script.m; Whole_Plant_Reactivity_Accident.m)
  mcp_f3 = mass_fn*Cp_f    (= 5.5019469141)    [Whole_Plant_Cool_Pump_Accident_script.m]    (also in Whole_Plant_Fert_Pump_Accident_script.m; Whole_Plant_Fuel_Pump_Accident.m; Whole_Plant_Fuel_Pump_Accident_script.m; Whole_Plant_Reactivity_Accident.m)
  mcp_f4 = mass_fn*Cp_f    (= 5.5019469141)    [Whole_Plant_Cool_Pump_Accident_script.m]    (also in Whole_Plant_Fert_Pump_Accident_script.m; Whole_Plant_Fuel_Pump_Accident.m; Whole_Plant_Fuel_Pump_Accident_script.m; Whole_Plant_Reactivity_Accident.m)
  mcp_g1 = (mass_grap*Cp_g)*K_fuel/2    (= 32.9814988203)    [Whole_Plant_Cool_Pump_Accident_script.m]    (also in Whole_Plant_Fert_Pump_Accident_script.m; Whole_Plant_Fuel_Pump_Accident.m; Whole_Plant_Fuel_Pump_Accident_script.m; Whole_Plant_Reactivity_Accident.m)
  mcp_g2 = mcp_g1    (= 32.9814988203)    [Whole_Plant_Cool_Pump_Accident_script.m]    (also in Whole_Plant_Fert_Pump_Accident_script.m; Whole_Plant_Fuel_Pump_Accident.m; Whole_Plant_Fuel_Pump_Accident_script.m; Whole_Plant_Reactivity_Accident.m)
  mcp_g3 = (mass_grap*Cp_g)*(1-K_fuel)    (= 8.15273004546)    [Whole_Plant_Cool_Pump_Accident_script.m]    (also in Whole_Plant_Fert_Pump_Accident_script.m; Whole_Plant_Fuel_Pump_Accident.m; Whole_Plant_Fuel_Pump_Accident_script.m; Whole_Plant_Reactivity_Accident.m)
  mcp_p_bhx1 = mp_bhx1*Cp_b    [Whole_Plant_Cool_Pump_Accident_script.m]    (also in Whole_Plant_Fert_Pump_Accident_script.m; Whole_Plant_Fuel_Pump_Accident.m; Whole_Plant_Fuel_Pump_Accident_script.m; Whole_Plant_Reactivity_Accident.m)
  mcp_p_bhx2 = mp_bhx2*Cp_b    [Whole_Plant_Cool_Pump_Accident_script.m]    (also in Whole_Plant_Fert_Pump_Accident_script.m; Whole_Plant_Fuel_Pump_Accident.m; Whole_Plant_Fuel_Pump_Accident_script.m; Whole_Plant_Reactivity_Accident.m)
  mcp_p_bhx3 = mp_bhx3*Cp_b    [Whole_Plant_Cool_Pump_Accident_script.m]    (also in Whole_Plant_Fert_Pump_Accident_script.m; Whole_Plant_Fuel_Pump_Accident.m; Whole_Plant_Fuel_Pump_Accident_script.m; Whole_Plant_Reactivity_Accident.m)
  ... (+213 more)
undefined symbols (not defined in the file or in its folder): C0, H_con_table, H_convap_table, H_rh_table, H_rh_table1, H_rh_table2, H_rhvap_table, H_s_table, H_table, P_con_table, P_nc_table, P_rh_table, P_rh_table1, pres_table, rho_rh_table, rho_table, SV_nc_table, SVf_nc_table, temp_table
(part 3 of 13)

== system MSBR_Plant/Nuclear Steam Supply System (NSSS)/MSBR ==
  In Bus Element2 : Inport  PortName=Core Inlet  Element=Fuel Heat Transfer Fraction
  In Bus Element : Inport  PortName=Core Inlet  Element=Hx Fuel Outlet Temp
  In Bus Element1 : Inport  PortName=Core Inlet  Element=Fuel Flow Fraction
  In Bus Element4 : Inport  PortName=Core Inlet  Element=Hx Blanket Outlet Temp
  In Bus Element5 : Inport  PortName=Core Inlet  Element=Blanket Flow Fraction
  In Bus Element3 : Inport  PortName=Core Inlet  Element=Blanket Heat Transfer Fraction
  Blanket Core to HX Delay : VariableTransportDelay  MaximumDelay=10000000  InitialOutput=T0_b2
  CORE HEAT TRANSFER : Subsystem
  Constant : Constant  Value=tau_c_fehx
  Constant1 : Constant  Value=tau_c_fhx
  Divide : Product  Inputs=*/
  Divide1 : Product  Inputs=*/
  Fuel Core to HX Delay : VariableTransportDelay  MaximumDelay=10000000  InitialOutput=T0_f4
  PKE SOLVER : Subsystem
  REACTIVITY : Subsystem
  Selector : Selector  InputPortWidth=9  IndexOptions=Index vector (dialog)  Indices=[6]  OutputSizes=1
  Selector1 : Selector  InputPortWidth=9  IndexOptions=Index vector (dialog)  Indices=[9]  OutputSizes=1
  XENON EFFECT ON REACTIVITY : Subsystem
  Bus Element Out1 : Outport  PortName=Fuel Core Outlet Temp  Element=Fuel Salt Temperature
  Out Bus Element : Outport  Port=2  PortName=Blanket Core Outlet Temp  Element=Blanket Salt Temperature
  wires:
  PKE SOLVER/1(Core Power (Frac)) -> [Core_Power_Frac_or_Neutron_Density_Frac]
  [Core_Power_Frac_or_Neutron_Density_Frac] -> CORE HEAT TRANSFER/1(Core Power (Frac))
  Selector/1 -> Fuel Core to HX Delay/1
  Selector1/1 -> Blanket Core to HX Delay/1
  CORE HEAT TRANSFER/1(Core Temperatures) -> [Core_Temps_out], Selector1/1, Selector/1
  [Core_Temps_out] -> REACTIVITY/1(Core Temperatures)
  In Bus Element/1 -> [Tf_in]
  In Bus Element2/1 -> [fuel_hA_frac]
  In Bus Element1/1 -> [fuel_flow_frac]
  In Bus Element3/1 -> [blanket_hA_frac]
  In Bus Element5/1 -> [blanket_flow_frac]
  In Bus Element4/1 -> [Tb_in]
  [Tf_in] -> CORE HEAT TRANSFER/2(Fuel Inlet Temperature)
  [Tb_in] -> CORE HEAT TRANSFER/3(Blanket Inlet Temperature)
  [fuel_flow_frac] -> CORE HEAT TRANSFER/4(Fuel Flow Fraction)
  [fuel_hA_frac] -> CORE HEAT TRANSFER/5(Fuel Heat Transfer Fraction)
  [blanket_flow_frac] -> CORE HEAT TRANSFER/6(Blanket Flow Fraction)
  [blanket_hA_frac] -> CORE HEAT TRANSFER/7(Blanket Heat Transfer Fraction)
  [fuel_flow_frac] -> PKE SOLVER/2(Fuel Flow Fraction)
  REACTIVITY/1(Total Reactivity Feedback) -> [rho_tot]
  [rho_tot] -> PKE SOLVER/1(Reactivity Feedback)
  XENON EFFECT ON REACTIVITY/1(drho_Xe) -> [drho_Xe]
  [drho_Xe] -> REACTIVITY/2(Xenon Reactivity)
  [Core_Power_Frac_or_Neutron_Density_Frac] -> XENON EFFECT ON REACTIVITY/1(Core Power (Frac))
  [fuel_flow_frac] -> Divide1/2
  Divide1/1 -> Fuel Core to HX Delay/2
  Fuel Core to HX Delay/1 -> Bus Element Out1/1
  [blanket_flow_frac] -> Divide/2
  Divide/1 -> Blanket Core to HX Delay/2
  Blanket Core to HX Delay/1 -> Out Bus Element/1
  Constant/1 -> Divide/1
  Constant1/1 -> Divide1/1

== system MSBR_Plant/Nuclear Steam Supply System (NSSS)/Once-Through Steam Generator (OTSG) ==
  Bus Element In2 : Inport  PortName=Feedwater  Element=Feedwater Temp
  Bus Element In5 : Inport  PortName=Feedwater  Element=Feedwater Flow
  Bus Element In1 : Inport  Port=2  PortName=Coolant Salt Inlet  Element=Coolant Outlet Temp
  Bus Element In3 : Inport  Port=2  PortName=Coolant Salt Inlet  Element=Coolant Flow Fraction
  Bus Element In4 : Inport  Port=2  PortName=Coolant Salt Inlet  Element=Coolant Heat Transfer Fraction
  Constant : Constant  Value=W_p0
  Constant4 : Constant  Value=P_set
  Display{12,14..15,47} (4 alike) : Display
  ONCE-THROUGH STEAM GENERATOR : Subsystem
  Product : Product
  Scope{4..7} (4 alike) : Scope
  Out Bus Element : Outport  PortName=NSSS Output  Element=Steam Temperature
  Out Bus Element1 : Outport  PortName=NSSS Output  Element=Steam Pressure
  Out Bus Element2 : Outport  PortName=NSSS Output  Element=Steam Flow Rate
  Out Bus Element3 : Outport  Port=2  PortName=Coolant Salt OTSG Outlet  Element=Coolant Salt Temperature
  wires:
  ONCE-THROUGH STEAM GENERATOR/1(Steam Temperature) -> Scope4/1, Display12/1, Out Bus Element/1, [T_steam_OTSG]
  ONCE-THROUGH STEAM GENERATOR/2(Coolant Salt Outlet Temperature) -> Out Bus Element3/1, Scope5/1, Display47/1
  Bus Element In3/1 -> Product/1
  ONCE-THROUGH STEAM GENERATOR/3(Steam Pressure) -> Out Bus Element1/1, Scope7/1, [P_steam_OTSG], Display14/1
  Constant4/1 -> ONCE-THROUGH STEAM GENERATOR/6(Pressure Set Point)
  ONCE-THROUGH STEAM GENERATOR/4(Steam Flow Rate) -> Scope6/1, Out Bus Element2/1, [steam_flow_OTSG], Display15/1
  Bus Element In1/1 -> ONCE-THROUGH STEAM GENERATOR/1(Coolant Salt Inlet Temp)
  Constant/1 -> Product/2
  Product/1 -> ONCE-THROUGH STEAM GENERATOR/3(Coolant Salt Flow Rate)
  Bus Element In4/1 -> ONCE-THROUGH STEAM GENERATOR/4(Coolant Salt Heat Transfer Frac)
  Bus Element In2/1 -> ONCE-THROUGH STEAM GENERATOR/2(Feedwater Inlet Temp)
  Bus Element In5/1 -> ONCE-THROUGH STEAM GENERATOR/5(Feedwater Flow Rate)

== system MSBR_Plant/Nuclear Steam Supply System (NSSS)/Primary Heat Exchanger Loops (Blanket and Fuel Salt HXs) ==
  In Bus Element2 : Inport  PortName=Fuel Salt Pump Input  Element=Flow and hA Frac
  In Bus Element5 : Inport  Port=2  PortName=Blanket Salt Pump Input  Element=Flow and hA Frac
  In Bus Element : Inport  Port=3  PortName=Fuel Salt Temp HX Inlet  Element=Fuel Salt Temperature
  In Bus Element3 : Inport  Port=4  PortName=Blanket Salt Temp HX Inlet  Element=Blanket Salt Temperature
  Bus Element In6 : Inport  Port=5  PortName=Coolant Salt Pump Input  Element=Flow and hA Frac
  In Bus Element1 : Inport  Port=6  PortName=Coolant Salt Temp HX Inlet  Element=Coolant Salt Temperature
  1-D Lookup Table1 : Lookup_n-D  NumberOfTableDimensions=1  BreakpointsForDimension1=xdat  Table=ydat  InternalRulePriority=Speed  RndMeth=Simplest  InputSameDT=on
  1-D Lookup Table2 : Lookup_n-D  NumberOfTableDimensions=1  BreakpointsForDimension1=xdat  Table=ydat  InternalRulePriority=Speed  RndMeth=Simplest  InputSameDT=on
  1-D Lookup Table3 : Lookup_n-D  NumberOfTableDimensions=1  BreakpointsForDimension1=xdatc  Table=ydatc  InternalRulePriority=Speed  RndMeth=Simplest  InputSameDT=on
  Blanket Pre Core Mixing : Subsystem
  Coolant Mix Temps : Scope
  Coolant Pre-BoP Mixing : Subsystem
  Demux : Demux  Outputs=8
  Demux1 : Demux  Outputs=8
  Demux2 : Demux  Outputs=8
  Fertile Mix Temps : Scope
  Fuel Mix Temps : Scope
  Fuel Pre Core Mixing : Subsystem
  HEAT EXCHANGER LOOP 1 : Subsystem
  HEAT EXCHANGER LOOP 2 : Subsystem
  HEAT EXCHANGER LOOP 3 : Subsystem
  HEAT EXCHANGER LOOP 4 : Subsystem
  To Workspace : ToWorkspace  VariableName=Pre_Core_Fuel_hA_frac  SaveFormat=Timeseries  SampleTime=-1
  To Workspace1 : ToWorkspace  VariableName=Pre_Core_Fert_hA_frac  SaveFormat=Timeseries  SampleTime=-1
  To Workspace2 : ToWorkspace  VariableName=Pre_OTSG_cool_hA_frac  SaveFormat=Timeseries  SampleTime=-1
  Out Bus Element1 : Outport  VectorParamsAs1DForOutWhenUnconnected=off  PortName=Fuel & Blanket Salt Outlet  Element=Hx Fuel Outlet Temp
  Out Bus Element5 : Outport  VectorParamsAs1DForOutWhenUnconnected=off  PortName=Fuel & Blanket Salt Outlet  Element=Hx Blanket Outlet Temp
  Out Bus Element6 : Outport  VectorParamsAs1DForOutWhenUnconnected=off  PortName=Fuel & Blanket Salt Outlet  Element=Fuel Flow Fraction
  Out Bus Element7 : Outport  VectorParamsAs1DForOutWhenUnconnected=off  PortName=Fuel & Blanket Salt Outlet  Element=Fuel Heat Transfer Fraction
  Out Bus Element2 : Outport  VectorParamsAs1DForOutWhenUnconnected=off  PortName=Fuel & Blanket Salt Outlet  Element=Blanket Flow Fraction
  Out Bus Element3 : Outport  VectorParamsAs1DForOutWhenUnconnected=off  PortName=Fuel & Blanket Salt Outlet  Element=Blanket Heat Transfer Fraction
  Out Bus Element10 : Outport  Port=2  PortName=Coolant Salt Outlet  Element=Coolant Outlet Temp
  Out Bus Element11 : Outport  Port=2  PortName=Coolant Salt Outlet  Element=Coolant Flow Fraction
  Out Bus Element12 : Outport  Port=2  PortName=Coolant Salt Outlet  Element=Coolant Heat Transfer Fraction
  wires:
  In Bus Element/1 -> [Tf_in]
  In Bus Element1/1 -> [Ts_in]
  In Bus Element3/1 -> [Tb_in]
  [fuel_hA_frac1] -> HEAT EXCHANGER LOOP 1/3(Fuel Heat Transfer Fraction)
  [fuel_flow_frac1] -> HEAT EXCHANGER LOOP 1/2(Fuel Flow)
  [Tf_out2] -> Fuel Pre Core Mixing/3(Tf_out2)
  [Ts_in] -> HEAT EXCHANGER LOOP 1/7(Coolant HX Inlet Temperature)
  [Tf_out3] -> Fuel Pre Core Mixing/5(Tf_out3)
  HEAT EXCHANGER LOOP 1/3(HX1 Coolant Outlet) -> [Ts_out1]
  [Tf_out1] -> Fuel Pre Core Mixing/1(Tf_out1)
  HEAT EXCHANGER LOOP 1/1(HX1 Fuel Outlet) -> [Tf_out1]
  [Tf_in] -> HEAT EXCHANGER LOOP 1/1(Fuel HX Inlet Temperature)
  [fuel_flow_frac3] -> Fuel Pre Core Mixing/6(Fuel Flow 3)
  [fuel_flow_frac2] -> Fuel Pre Core Mixing/4(Fuel Flow 2)
  Fuel Pre Core Mixing/1(Tf_out) -> Fuel Mix Temps/1, Out Bus Element1/1
  [fuel_flow_frac1] -> Fuel Pre Core Mixing/2(Fuel Flow 1)
  [Tb_in] -> HEAT EXCHANGER LOOP 1/4(Blanket HX Inlet Temperature)
  [blank_hA_frac1] -> HEAT EXCHANGER LOOP 1/6(Blanket Heat Transfer Fraction)
  [blank_flow_frac1] -> HEAT EXCHANGER LOOP 1/5(Blanket Flow)
  HEAT EXCHANGER LOOP 1/2(HX1 Blanket Outlet) -> [Tb_out1]
  HEAT EXCHANGER LOOP 2/2(HX2 Blanket Outlet) -> [Tb_out2]
  HEAT EXCHANGER LOOP 2/1(HX2 Fuel Outlet) -> [Tf_out2]
  [Tb_in] -> HEAT EXCHANGER LOOP 2/4(Blanket HX Inlet Temperature)
  [fuel_flow_frac2] -> HEAT EXCHANGER LOOP 2/2(Fuel Flow)
  [blank_hA_frac2] -> HEAT EXCHANGER LOOP 2/6(Blanket Heat Transfer Fraction)
  [blank_flow_frac2] -> HEAT EXCHANGER LOOP 2/5(Blanket Flow)
  [Tf_in] -> HEAT EXCHANGER LOOP 2/1(Fuel HX Inlet Temperature)
  HEAT EXCHANGER LOOP 2/3(HX2 Coolant Outlet) -> [Ts_out2]
  [Ts_in] -> HEAT EXCHANGER LOOP 2/7(Coolant HX Inlet Temperature)
  [fuel_hA_frac2] -> HEAT EXCHANGER LOOP 2/3(Fuel Heat Transfer Fraction)
  [fuel_hA_frac3] -> HEAT EXCHANGER LOOP 3/3(Fuel Heat Transfer Fraction)
  HEAT EXCHANGER LOOP 3/1(HX3 Fuel Outlet) -> [Tf_out3]
  [Tb_in] -> HEAT EXCHANGER LOOP 3/4(Blanket HX Inlet Temperature)
  HEAT EXCHANGER LOOP 3/2(HX3 Blanket Outlet) -> [Tb_out3]
  [blank_hA_frac3] -> HEAT EXCHANGER LOOP 3/6(Blanket Heat Transfer Fraction)
  HEAT EXCHANGER LOOP 3/3(HX3 Coolant Outlet) -> [Ts_out3]
  [Tf_in] -> HEAT EXCHANGER LOOP 3/1(Fuel HX Inlet Temperature)
  [Ts_in] -> HEAT EXCHANGER LOOP 3/7(Coolant HX Inlet Temperature)
  [fuel_flow_frac3] -> HEAT EXCHANGER LOOP 3/2(Fuel Flow)
  [blank_flow_frac3] -> HEAT EXCHANGER LOOP 3/5(Blanket Flow)
  [fuel_hA_frac4] -> HEAT EXCHANGER LOOP 4/3(Fuel Heat Transfer Fraction)
  HEAT EXCHANGER LOOP 4/1(HX4 Fuel Outlet) -> [Tf_out4]
  [Tb_in] -> HEAT EXCHANGER LOOP 4/4(Blanket HX Inlet Temperature)
  HEAT EXCHANGER LOOP 4/2(HX4 Blanket Outlet) -> [Tb_out4]
  [blank_hA_frac4] -> HEAT EXCHANGER LOOP 4/6(Blanket Heat Transfer Fraction)
  HEAT EXCHANGER LOOP 4/3(HX4 Coolant Outlet) -> [Ts_out4]
  [Tf_in] -> HEAT EXCHANGER LOOP 4/1(Fuel HX Inlet Temperature)
  [Ts_in] -> HEAT EXCHANGER LOOP 4/7(Coolant HX Inlet Temperature)
  [fuel_flow_frac4] -> HEAT EXCHANGER LOOP 4/2(Fuel Flow)
  [blank_flow_frac4] -> HEAT EXCHANGER LOOP 4/5(Blanket Flow)
  [Tf_out4] -> Fuel Pre Core Mixing/7(Tf_out4)
  [fuel_flow_frac4] -> Fuel Pre Core Mixing/8(Fuel Flow 4)
  [blank_flow_frac4] -> Blanket Pre Core Mixing/8(Blanket Flow 4)
  [blank_flow_frac1] -> Blanket Pre Core Mixing/2(Blanket Flow 1)
  Blanket Pre Core Mixing/1(Tb_out) -> Fertile Mix Temps/1, Out Bus Element5/1
  [Tb_out2] -> Blanket Pre Core Mixing/3(Tb_out2)
  [Tb_out4] -> Blanket Pre Core Mixing/7(Tb_out4)
  [blank_flow_frac3] -> Blanket Pre Core Mixing/6(Blanket Flow 3)
  [Tb_out3] -> Blanket Pre Core Mixing/5(Tb_out3)
  [blank_flow_frac2] -> Blanket Pre Core Mixing/4(Blanket Flow 2)
  [Tb_out1] -> Blanket Pre Core Mixing/1(Tb_out1)
  Fuel Pre Core Mixing/2(Total Fuel Flow Frac) -> 1-D Lookup Table2/1, Out Bus Element6/1
  1-D Lookup Table2/1 -> To Workspace/1, Out Bus Element7/1
  Blanket Pre Core Mixing/2(Total Blanket Flow Frac) -> 1-D Lookup Table1/1, Out Bus Element2/1
  1-D Lookup Table1/1 -> To Workspace1/1, Out Bus Element3/1
  Coolant Pre-BoP Mixing/2(Total Coolant Flow Frac) -> Out Bus Element11/1, 1-D Lookup Table3/1
  [cool_flow_frac2] -> Coolant Pre-BoP Mixing/4(Coolant Flow 2)
  [cool_flow_frac3] -> Coolant Pre-BoP Mixing/6(Coolant Flow 3)
  [cool_flow_frac4] -> Coolant Pre-BoP Mixing/8(Coolant Flow 4)
  Coolant Pre-BoP Mixing/1(Ts_out) -> Coolant Mix Temps/1, Out Bus Element10/1
  [Ts_out2] -> Coolant Pre-BoP Mixing/3(Ts_out2)
  [Ts_out3] -> Coolant Pre-BoP Mixing/5(Ts_out3)
  [Ts_out1] -> Coolant Pre-BoP Mixing/1(Ts_out1)
  [Ts_out4] -> Coolant Pre-BoP Mixing/7(Ts_out4)
  [cool_flow_frac1] -> Coolant Pre-BoP Mixing/2(Coolant Flow 1)
  In Bus Element2/1 -> Demux/1
  Demux/1 -> [fuel_flow_frac1]
  Demux/2 -> [fuel_hA_frac1]
  Demux/3 -> [fuel_flow_frac2]
  Demux/4 -> [fuel_hA_frac2]
  Demux/5 -> [fuel_flow_frac3]
  Demux/6 -> [fuel_hA_frac3]
  Demux/7 -> [fuel_flow_frac4]
  Demux/8 -> [fuel_hA_frac4]
  In Bus Element5/1 -> Demux1/1
  Demux1/1 -> [blank_flow_frac1]
  Demux1/2 -> [blank_hA_frac1]
  Demux1/3 -> [blank_flow_frac2]
  Demux1/4 -> [blank_hA_frac2]
  Demux1/5 -> [blank_flow_frac3]
  Demux1/6 -> [blank_hA_frac3]
  Demux1/7 -> [blank_flow_frac4]
  Demux1/8 -> [blank_hA_frac4]
  Bus Element In6/1 -> Demux2/1
  Demux2/1 -> [cool_flow_frac1]
  Demux2/2 -> [cool_hA_frac1]
  Demux2/3 -> [cool_flow_frac2]
  Demux2/4 -> [cool_hA_frac2]
  Demux2/5 -> [cool_flow_frac3]
  Demux2/6 -> [cool_hA_frac3]
  Demux2/7 -> [cool_flow_frac4]
  Demux2/8 -> [cool_hA_frac4]
  [cool_flow_frac1] -> HEAT EXCHANGER LOOP 1/8(Coolant Flow Fraction)
  [cool_hA_frac1] -> HEAT EXCHANGER LOOP 1/9(Coolant hA Fraction)
  [cool_flow_frac2] -> HEAT EXCHANGER LOOP 2/8(Coolant Flow Fraction)
  [cool_hA_frac2] -> HEAT EXCHANGER LOOP 2/9(Coolant hA Fraction)
  [cool_flow_frac3] -> HEAT EXCHANGER LOOP 3/8(Coolant Flow Fraction)
  [cool_hA_frac3] -> HEAT EXCHANGER LOOP 3/9(Coolant hA Fraction)
  [cool_flow_frac4] -> HEAT EXCHANGER LOOP 4/8(Coolant Flow Fraction)
  [cool_hA_frac4] -> HEAT EXCHANGER LOOP 4/9(Coolant hA Fraction)
  1-D Lookup Table3/1 -> To Workspace2/1, Out Bus Element12/1

== system MSBR_Plant/Nuclear Steam Supply System (NSSS)/Primary Pumps (Blanket and Fuel Salt) ==
  Blanket Pump 1 : Subsystem
  Blanket Pump 2 : Subsystem
  Blanket Pump 3 : Subsystem
  Blanket Pump 4 : Subsystem
  Constant : Constant  Value=therm_conv_fuel
  Constant1 : Constant  Value=therm_conv_blank
  Constant2 : Constant  Value=tau_p_f
  Constant3 : Constant  Value=tau_p_b
  Constant4 : Constant  Value=trip_time_f
  Constant5 : Constant  Value=trip_time_b
  Demux{,1..5} (6 alike) : Demux
  Fuel Pump 1 : Subsystem
  Fuel Pump 2 : Subsystem
  Fuel Pump 3 : Subsystem
  Fuel Pump 4 : Subsystem
  Mux : Mux  Inputs=8
  Mux1 : Mux  Inputs=8
  Out Bus Element : Outport  PortName=Fuel Pumps  Element=Flow and hA Frac
  Out Bus Element1 : Outport  Port=2  PortName=Blanket Pumps  Element=Flow and hA Frac
  wires:
  Fuel Pump 1/1(Fuel Flow Fraction) -> Mux/1
  Fuel Pump 3/1(Fuel Flow Fraction) -> Mux/5
  Fuel Pump 3/2(Fuel Heat Transfer Fraction) -> Mux/6
  Mux/1 -> Out Bus Element/1
  Mux1/1 -> Out Bus Element1/1
  Fuel Pump 1/2(Fuel Heat Transfer Fraction) -> Mux/2
  Fuel Pump 2/1(Fuel Flow Fraction) -> Mux/3
  Fuel Pump 2/2(Fuel Heat Transfer Fraction) -> Mux/4
  Fuel Pump 4/1(Fuel Flow Fraction) -> Mux/7
  Fuel Pump 4/2(Fuel Heat Transfer Fraction) -> Mux/8
  Blanket Pump 1/1(Blanket Flow Fraction) -> Mux1/1
  Blanket Pump 1/2(Blanket Heat Transfer Fraction) -> Mux1/2
  Blanket Pump 2/1(Blanket Flow Fraction) -> Mux1/3
  Blanket Pump 2/2(Blanket Heat Transfer Fraction) -> Mux1/4
  Blanket Pump 3/1(Blanket Flow Fraction) -> Mux1/5
  Blanket Pump 3/2(Blanket Heat Transfer Fraction) -> Mux1/6
  Blanket Pump 4/1(Blanket Flow Fraction) -> Mux1/7
  Blanket Pump 4/2(Blanket Heat Transfer Fraction) -> Mux1/8
  Constant/1 -> Demux/1
  Constant2/1 -> Demux2/1
  Constant4/1 -> Demux4/1
  Demux2/1 -> Fuel Pump 1/1(Pump Decay Rate)
  Demux/1 -> Fuel Pump 1/2(Thermal Conv)
  Demux2/2 -> Fuel Pump 2/1(Pump Decay Rate)
  Demux2/3 -> Fuel Pump 3/1(Pump Decay Rate)
  Demux2/4 -> Fuel Pump 4/1(Pump Decay Rate)
  Demux/2 -> Fuel Pump 2/2(Thermal Conv)
  Demux/3 -> Fuel Pump 3/2(Thermal Conv)
  Demux/4 -> Fuel Pump 4/2(Thermal Conv)
  Demux4/1 -> Fuel Pump 1/3(Pump Trip Time)
  Demux4/2 -> Fuel Pump 2/3(Pump Trip Time)
  Demux4/3 -> Fuel Pump 3/3(Pump Trip Time)
  Demux4/4 -> Fuel Pump 4/3(Pump Trip Time)
  Demux3/1 -> Blanket Pump 1/1(Pump Decay Rate)
  Demux5/1 -> Blanket Pump 1/3(Pump Trip Time)
  Demux3/3 -> Blanket Pump 3/1(Pump Decay Rate)
  Demux1/3 -> Blanket Pump 3/2(Thermal Conv)
  Demux5/3 -> Blanket Pump 3/3(Pump Trip Time)
  Demux1/4 -> Blanket Pump 4/2(Thermal Conv)
  Demux1/2 -> Blanket Pump 2/2(Thermal Conv)
  Demux5/4 -> Blanket Pump 4/3(Pump Trip Time)
  Demux3/2 -> Blanket Pump 2/1(Pump Decay Rate)
  Constant5/1 -> Demux5/1
  Demux5/2 -> Blanket Pump 2/3(Pump Trip Time)
  Demux3/4 -> Blanket Pump 4/1(Pump Decay Rate)
  Demux1/1 -> Blanket Pump 1/2(Thermal Conv)
  Constant3/1 -> Demux3/1
  Constant1/1 -> Demux1/1

== system MSBR_Plant/Nuclear Steam Supply System (NSSS)/Coolant Salt Pumps/Coolant Pump 1 ==
  note: Exponentional Function that decays with time (beginning at pump trip time). Decay rate is determined by tau_p of the pump. Final fractonal value of flow through piping is the thermal conv.
  note: Note that it is possible to put in a step function for the pump to reduce flow rate at a specific time. It could simulate a pipe leak/break
  Pump Decay Rate : Inport
  Thermal Conv : Inport  Port=2
  Pump Trip Time : Inport  Port=3
  1-D Lookup Table1 : Lookup_n-D  NumberOfTableDimensions=1  BreakpointsForDimension1=xdatc  Table=ydatc  InternalRulePriority=Speed  RndMeth=Simplest  InputSameDT=on
  Clock1 : Clock
  Constant : Constant
  Constant1 : Constant  Value=-1
  Divide : Product  Inputs=*/
  Math Function : Math  SaturateOnIntegerOverflow=on
  Minus : Sum  Inputs=+-
  Minus1 : Sum  Inputs=+-
  Minus3 : Sum  Inputs=+-
  Product : Product
  Scope1 : Scope
  Switch1 : Switch  Criteria=u2 > Threshold
  Switch3 : Switch  Criteria=u2 > Threshold
  To Workspace : ToWorkspace  VariableName=cool_pump_1_flow_frac  SaveFormat=Timeseries  SampleTime=-1
  To Workspace1 : ToWorkspace  VariableName=cool_pump_1_hA_frac  SaveFormat=Timeseries  SampleTime=-1
  Coolant Flow Fraction : Outport  VectorParamsAs1DForOutWhenUnconnected=off
  Coolant Heat Transfer Fraction : Outport  Port=2  VectorParamsAs1DForOutWhenUnconnected=off
  wires:
  Pump Trip Time/1 -> Minus/1, Minus1/2
  Thermal Conv/1 -> Minus3/2, Switch3/3
  Pump Decay Rate/1 -> Divide/2
  Minus/1 -> Switch1/2
  Switch1/1 -> Switch3/1, Minus3/1
  Math Function/1 -> Switch1/3
  Clock1/1 -> Minus/2, Minus1/1
  Constant/1 -> Switch1/1
  Constant1/1 -> Divide/1
  Divide/1 -> Product/2
  Minus1/1 -> Product/1
  Product/1 -> Math Function/1
  Minus3/1 -> Switch3/2
  1-D Lookup Table1/1 -> To Workspace1/1, Coolant Heat Transfer Fraction/1
  Switch3/1 -> To Workspace/1, Coolant Flow Fraction/1, Scope1/1, 1-D Lookup Table1/1

== system MSBR_Plant/Nuclear Steam Supply System (NSSS)/Coolant Salt Pumps/Coolant Pump 2 ==
  note: Note that it is possible to put in a step function for the pump to reduce flow rate at a specific time. It could simulate a pipe leak/break
  note: Exponentional Function that decays with time (beginning at pump trip time). Decay rate is determined by tau_p of the pump. Final fractonal value of flow through piping is the thermal conv.
  Pump Decay Rate : Inport
  Thermal Conv : Inport  Port=2
  Pump Trip Time : Inport  Port=3
  1-D Lookup Table1 : Lookup_n-D  NumberOfTableDimensions=1  BreakpointsForDimension1=xdatc  Table=ydatc  InternalRulePriority=Speed  RndMeth=Simplest  InputSameDT=on
  Clock1 : Clock
  Constant : Constant
  Constant1 : Constant  Value=-1
  Divide : Product  Inputs=*/
  Math Function : Math  SaturateOnIntegerOverflow=on
  Minus : Sum  Inputs=+-
  Minus1 : Sum  Inputs=+-
  Minus3 : Sum  Inputs=+-
  Product : Product
  Scope1 : Scope
  Switch1 : Switch  Criteria=u2 > Threshold
  Switch3 : Switch  Criteria=u2 > Threshold
  To Workspace : ToWorkspace  VariableName=cool_pump_2_flow_frac  SaveFormat=Timeseries  SampleTime=-1
  To Workspace1 : ToWorkspace  VariableName=cool_pump_2_hA_frac  SaveFormat=Timeseries  SampleTime=-1
  Coolant Flow Fraction : Outport  VectorParamsAs1DForOutWhenUnconnected=off
  Coolant Heat Transfer Fraction : Outport  Port=2  VectorParamsAs1DForOutWhenUnconnected=off
  wires:
  Minus3/1 -> Switch3/2
  Product/1 -> Math Function/1
  Minus1/1 -> Product/1
  Divide/1 -> Product/2
  Constant1/1 -> Divide/1
  Constant/1 -> Switch1/1
  Clock1/1 -> Minus1/1, Minus/2
  Math Function/1 -> Switch1/3
  Switch1/1 -> Minus3/1, Switch3/1
  Minus/1 -> Switch1/2
  Pump Decay Rate/1 -> Divide/2
  Thermal Conv/1 -> Switch3/3, Minus3/2
  Pump Trip Time/1 -> Minus1/2, Minus/1
  Switch3/1 -> 1-D Lookup Table1/1, Scope1/1, To Workspace/1, Coolant Flow Fraction/1
  1-D Lookup Table1/1 -> To Workspace1/1, Coolant Heat Transfer Fraction/1

== system MSBR_Plant/Nuclear Steam Supply System (NSSS)/Coolant Salt Pumps/Coolant Pump 3 ==
  note: Exponentional Function that decays with time (beginning at pump trip time). Decay rate is determined by tau_p of the pump. Final fractonal value of flow through piping is the thermal conv.
  note: Note that it is possible to put in a step function for the pump to reduce flow rate at a specific time. It could simulate a pipe leak/break
  Pump Decay Rate : Inport
  Thermal Conv : Inport  Port=2
  Pump Trip Time : Inport  Port=3
  1-D Lookup Table1 : Lookup_n-D  NumberOfTableDimensions=1  BreakpointsForDimension1=xdatc  Table=ydatc  InternalRulePriority=Speed  RndMeth=Simplest  InputSameDT=on
  Clock1 : Clock
  Constant : Constant
  Constant1 : Constant  Value=-1
  Divide : Product  Inputs=*/
  Math Function : Math  SaturateOnIntegerOverflow=on
  Minus : Sum  Inputs=+-
  Minus1 : Sum  Inputs=+-
  Minus3 : Sum  Inputs=+-
  Product : Product
  Scope1 : Scope
  Switch1 : Switch  Criteria=u2 > Threshold
  Switch3 : Switch  Criteria=u2 > Threshold
  To Workspace : ToWorkspace  VariableName=cool_pump_3_flow_frac  SaveFormat=Timeseries  SampleTime=-1
  To Workspace1 : ToWorkspace  VariableName=cool_pump_3_hA_frac  SaveFormat=Timeseries  SampleTime=-1
  Coolant Flow Fraction : Outport  VectorParamsAs1DForOutWhenUnconnected=off
  Coolant Heat Transfer Fraction : Outport  Port=2  VectorParamsAs1DForOutWhenUnconnected=off
  wires:
  Pump Trip Time/1 -> Minus/1, Minus1/2
  Thermal Conv/1 -> Minus3/2, Switch3/3
  Pump Decay Rate/1 -> Divide/2
  Minus/1 -> Switch1/2
  Switch1/1 -> Switch3/1, Minus3/1
  Math Function/1 -> Switch1/3
  Clock1/1 -> Minus/2, Minus1/1
  Constant/1 -> Switch1/1
  Constant1/1 -> Divide/1
  Divide/1 -> Product/2
  Minus1/1 -> Product/1
  Product/1 -> Math Function/1
  Minus3/1 -> Switch3/2
  Switch3/1 -> To Workspace/1, Coolant Flow Fraction/1, Scope1/1, 1-D Lookup Table1/1
  1-D Lookup Table1/1 -> To Workspace1/1, Coolant Heat Transfer Fraction/1
